simulink model "One_Leg_Robot"  (Simulink 7.3)
settings: Solver=ode15s  StartTime=0.0  StopTime=inf  RelTol=1e-3
PreLoadFcn:
  | init_hopper
PostLoadFcn:
  | vrmfunc('FnOpen', [bdroot, '/Data Display and Analysis/VR Sink']);
undefined symbols (not defined in the file or in its folder): body, ctrl, ground, leg, sigbuilder_block, Traj
libraries: mblibv1 x27, simulink x4
(part 2 of 2)

== system One_Leg_Robot/Robot/Leg Tip and Contact Dynamics/Contact Force/Force Law/Zero Force ==
  Action Port : ActionPort  ActionType=else
  Zero Force : Constant  Value=[0;0;0]  OutDataType=sfix(16)  OutScaling=2^0
  force : Outport  OutDataType=sfix(16)  OutScaling=2^0  InitialOutput=0
  wires:
  Zero Force/1 -> force/1

== system One_Leg_Robot/Robot/Leg Tip and Contact Dynamics/Contact Force/Force Law/Contact Force/Store Initial Value ==
  In1 : Inport  OutDataType=sfix(16)  OutScaling=2^0
  Enable : EnablePort
  Set Y=0 : Gain  Gain=[1 0 1]  ParameterDataType=sfix(16)  ParameterScaling=2^0  OutDataType=sfix(16)  OutScaling=2^0  SaturateOnIntegerOverflow=on  OutDataTypeStr=Inherit: Same as input  ParamDataTypeStr=Inherit: Same as input
  Out1 : Outport  OutDataType=sfix(16)  OutScaling=2^0
  wires:
  Set Y=0/1 -> Out1/1
  In1/1 -> Set Y=0/1
